simulink model "LTI_test"  (R2016b)
settings: Solver=VariableStepAuto  StartTime=0.0  StopTime=10.0  RelTol=1e-3
undefined symbols (not defined in the file): A, A1, B, B1, C, C1, D, D1, x0, x1
settings Model: Creator=arthus  LastModifiedBy=arthus

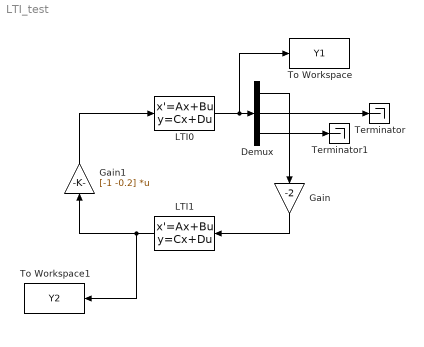
== system LTI_test ==
  Demux : Demux  Outputs=3
  Gain : Gain  Gain=-2
  Gain1 : Gain  Gain=[-1 -0.2]  Multiplication=Matrix(K*u)
  LTI0 : StateSpace  A=A  B=B  C=C  D=D  X0=x0
  LTI1 : StateSpace  A=A1  B=B1  C=C1  D=D1  X0=x1
  Terminator : Terminator
  Terminator1 : Terminator
  To Workspace : ToWorkspace  VariableName=Y1  SaveFormat=Timeseries  SampleTime=-1
  To Workspace1 : ToWorkspace  VariableName=Y2  SaveFormat=Timeseries  SampleTime=-1
  wires:
  Gain/1 -> LTI1/1
  LTI0/1 -> To Workspace/1, Demux/1
  Demux/1 -> Gain/1
  Demux/2 -> Terminator/1
  Demux/3 -> Terminator1/1
  LTI1/1 -> Gain1/1, To Workspace1/1
  Gain1/1 -> LTI0/1
